simulink model "parfait"  (Simulink 6.0)
settings: Solver=ode23  StartTime=0.0  StopTime=10.0  FixedStep=1e-4  RelTol=1e-3
libraries: simulink x9, aerolibutil x5, aerolibtransform2 x2, mblibv1 x1, aerolib6dof2 x1, vrlib x1
settings Model: LastModifiedBy=sebastien

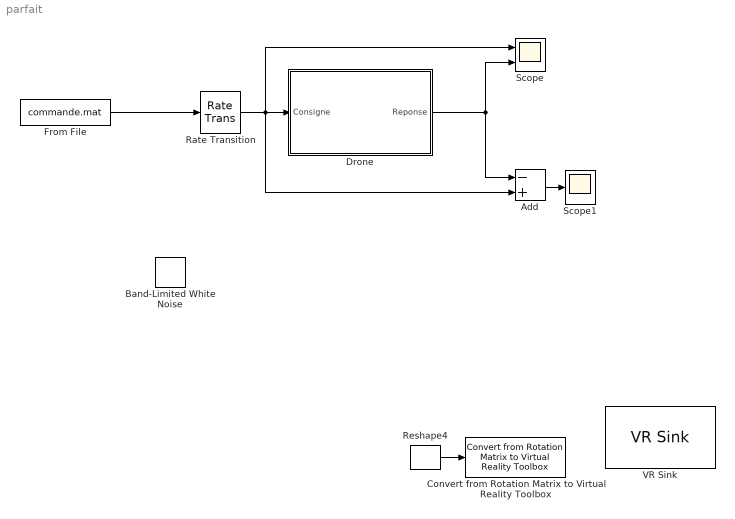
== system parfait ==
  Add : Sum  Inputs=-+  OutScaling=2^-10
  Band-Limited White Noise : simulink/Sources/Band-Limited White Noise  Cov=0.2*[1 1 1 1 1 1]  Ts=1  seed=[23341 3456 665332 234343 232324 45799]
  Convert from Rotation Matrix to Virtual Reality Toolbox : mblibv1/Utilities/Convert from Rotation Matrix to Virtual Reality Toolbox  Tag=Pose2VR
  Drone : Subsystem
  From File : FromFile  FileName=commande.mat  SampleTime=0
  Rate Transition : RateTransition
  Reshape4 : simulink/Math Operations/Reshape  OutputDimensionality=1-D array  OutputDimensions=[1,1]
  Scope : Scope  NumInputPorts=2
      settings: YMin=0~-0.2  YMax=2~2.1
  Scope1 : Scope
  VR Sink : vrlib/VR Sink  SampleTime=0.1  ViewEnable=on  RemoteChange=off  RemoteView=on  FieldsWritten=Drone.center.3.1.double#Drone.rotation.4.1.double  WorldFileName=drone2.WRL  AutoView=off  FigureProperties={}
  wires:
  Reshape4/1 -> Convert from Rotation Matrix to Virtual Reality Toolbox/1
  From File/1 -> Rate Transition/1
  Drone/1(Reponse) -> Scope/2, Add/1
  Rate Transition/1 -> Drone/1(Consigne), Scope/1, Add/2
  Add/1 -> Scope1/1

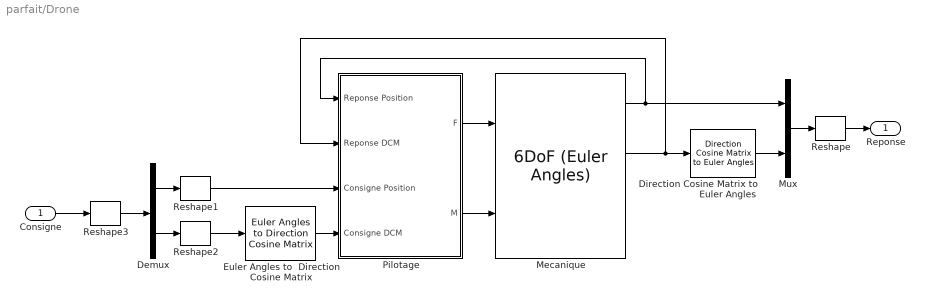
== system parfait/Drone ==
  Consigne : Inport  Port=1  LatchInput=off
  Demux : Demux  Outputs=2
  Direction Cosine Matrix to Euler Angles : aerolibtransform2/Direction Cosine Matrix to Euler Angles
  Euler Angles to  Direction Cosine Matrix : aerolibtransform2/Euler Angles to  Direction Cosine Matrix
  Mecanique : aerolib6dof2/6DoF (Euler Angles)  units=Metric (MKS)  mtype=Fixed  rep=Quaternion  xme_0=[0 0 0]  Vm_0=[0 0 0]  eul_0=[0 0 0]  pm_0=[1 2 4]  mass_0=1.0  mass_e=0  mass_f=0  inertia=eye(3)  inertia_e=eye(3)  inertia_f=eye(3)  k_quat=1.0
  Mux : Mux  Inputs=2
  Pilotage : Subsystem
  Reshape{,1..3} (4 alike) : simulink/Math Operations/Reshape  OutputDimensionality=1-D array  OutputDimensions=[1,1]
  Reponse : Outport
  wires:
  Pilotage/1(F) -> Mecanique/1
  Mecanique/2 -> Pilotage/1(Reponse Position), Mux/1
  Mecanique/4 -> Pilotage/2(Reponse DCM), Direction Cosine Matrix to Euler Angles/1
  Euler Angles to  Direction Cosine Matrix/1 -> Pilotage/4(Consigne DCM)
  Consigne/1 -> Reshape3/1
  Direction Cosine Matrix to Euler Angles/1 -> Mux/2
  Mux/1 -> Reshape/1
  Reshape1/1 -> Pilotage/3(Consigne Position)
  Reshape2/1 -> Euler Angles to  Direction Cosine Matrix/1
  Reshape3/1 -> Demux/1
  Pilotage/2(M) -> Mecanique/2
  Demux/1 -> Reshape1/1
  Demux/2 -> Reshape2/1
  Reshape/1 -> Reponse/1

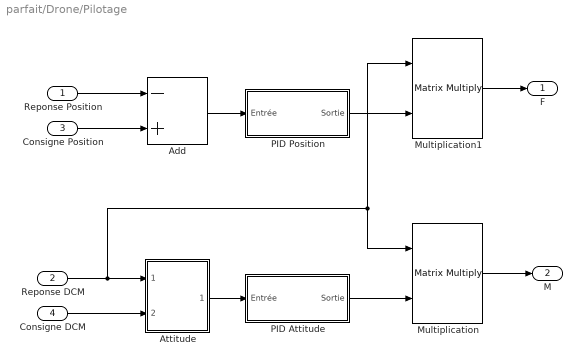
== system parfait/Drone/Pilotage ==
  Reponse Position : Inport  Port=1  LatchInput=off
  Reponse DCM : Inport  Port=2  LatchInput=off
  Consigne Position : Inport  Port=3  LatchInput=off
  Consigne DCM : Inport  Port=4  LatchInput=off
  Add : Sum  Inputs=-+  OutScaling=2^-10  InputSameDT=on
  Attitude : Subsystem
  Multiplication : Product  Inputs=**  Multiplication=Matrix(*)  OutScaling=2^-10
  Multiplication1 : Product  Inputs=**  Multiplication=Matrix(*)  OutScaling=2^-10
  PID Attitude : Subsystem  mask{kp=1000, ki=0.1, kd=0.05, kdd=0}
  PID Position : Subsystem  mask{kp=1000, ki=0.1, kd=0.05, kdd=0}
  F : Outport
  M : Outport  Port=2
  wires:
  Reponse Position/1 -> Add/1
  Consigne Position/1 -> Add/2
  Add/1 -> PID Position/1(Entrée)
  Consigne DCM/1 -> Attitude/2(Consigne)
  Reponse DCM/1 -> Attitude/1(Reponse), Multiplication1/1, Multiplication/1
  Attitude/1(Commande) -> PID Attitude/1(Entrée)
  PID Attitude/1(Sortie) -> Multiplication/2
  PID Position/1(Sortie) -> Multiplication1/2
  Multiplication/1 -> M/1
  Multiplication1/1 -> F/1

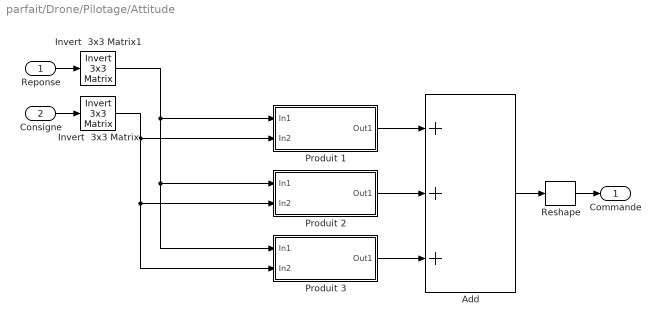
== system parfait/Drone/Pilotage/Attitude ==
  Reponse : Inport  Port=1  LatchInput=off
  Consigne : Inport  Port=2  LatchInput=off
  Add : Sum  Inputs=+++  OutScaling=2^-10
  Invert  3x3 Matrix : aerolibutil/Invert  3x3 Matrix
  Invert  3x3 Matrix1 : aerolibutil/Invert  3x3 Matrix
  Produit 1 : Subsystem  mask{a=[1 0 0]}
      mask prompts: a "Vecteur de reference"
      mask Display: fprintf('Vecteur (%d,%d,%d)', a(1),a(2),a(3))
  Produit 2 : Subsystem  mask{a=[0 1 0]}
      mask prompts: a "Vecteur de reference"
      mask Display: fprintf('Vecteur (%d,%d,%d)', a(1),a(2),a(3))
  Produit 3 : Subsystem  mask{a=[0 0 1]}
      mask prompts: a "Vecteur de reference"
      mask Display: fprintf('Vecteur (%d,%d,%d)', a(1),a(2),a(3))
  Reshape : simulink/Math Operations/Reshape  OutputDimensionality=1-D array  OutputDimensions=[1,1]
  Commande : Outport
  wires:
  Reponse/1 -> Invert  3x3 Matrix1/1
  Consigne/1 -> Invert  3x3 Matrix/1
  Produit 1/1(Out1) -> Add/1
  Produit 2/1(Out1) -> Add/2
  Produit 3/1(Out1) -> Add/3
  Invert  3x3 Matrix/1 -> Produit 1/2(In2), Produit 2/2(In2), Produit 3/2(In2)
  Invert  3x3 Matrix1/1 -> Produit 1/1(In1), Produit 2/1(In1), Produit 3/1(In1)
  Add/1 -> Reshape/1
  Reshape/1 -> Commande/1

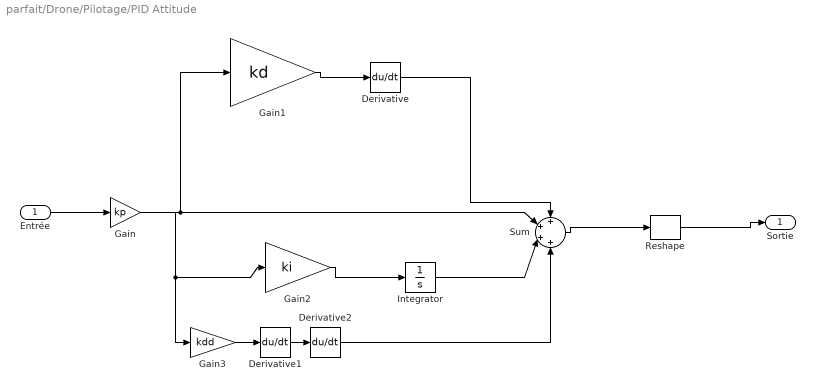
== system parfait/Drone/Pilotage/PID Attitude ==
  Entrée : Inport  Port=1  LatchInput=off
  Derivative : Derivative
  Derivative1 : Derivative
  Derivative2 : Derivative
  Gain : Gain  Gain=kp
  Gain1 : Gain  Gain=kd
  Gain2 : Gain  Gain=ki
  Gain3 : Gain  Gain=kdd
  Integrator : Integrator
  Reshape : simulink/Math Operations/Reshape  OutputDimensionality=1-D array  OutputDimensions=[1,1]
  Sum : Sum  Inputs=++++
  Sortie : Outport
      settings: BusObject=perturbations
  wires:
  Entrée/1 -> Gain/1
  Gain/1 -> Sum/2, Gain1/1, Gain2/1, Gain3/1
  Derivative/1 -> Sum/1
  Integrator/1 -> Sum/3
  Gain2/1 -> Integrator/1
  Gain1/1 -> Derivative/1
  Sum/1 -> Reshape/1
  Gain3/1 -> Derivative1/1
  Derivative1/1 -> Derivative2/1
  Derivative2/1 -> Sum/4
  Reshape/1 -> Sortie/1

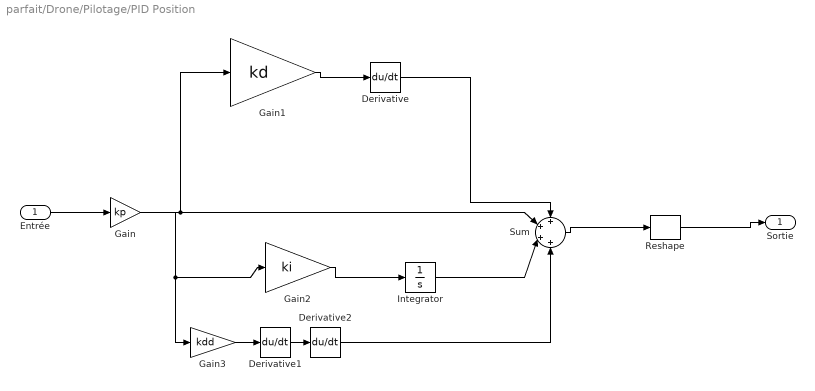
== system parfait/Drone/Pilotage/PID Position ==
  Entrée : Inport  Port=1  LatchInput=off
  Derivative : Derivative
  Derivative1 : Derivative
  Derivative2 : Derivative
  Gain : Gain  Gain=kp
  Gain1 : Gain  Gain=kd
  Gain2 : Gain  Gain=ki
  Gain3 : Gain  Gain=kdd
  Integrator : Integrator
  Reshape : simulink/Math Operations/Reshape  OutputDimensionality=1-D array  OutputDimensions=[1,1]
  Sum : Sum  Inputs=++++
  Sortie : Outport
      settings: BusObject=perturbations
  wires:
  Entrée/1 -> Gain/1
  Gain/1 -> Sum/2, Gain1/1, Gain2/1, Gain3/1
  Derivative/1 -> Sum/1
  Integrator/1 -> Sum/3
  Gain2/1 -> Integrator/1
  Gain1/1 -> Derivative/1
  Sum/1 -> Reshape/1
  Gain3/1 -> Derivative1/1
  Derivative1/1 -> Derivative2/1
  Derivative2/1 -> Sum/4
  Reshape/1 -> Sortie/1

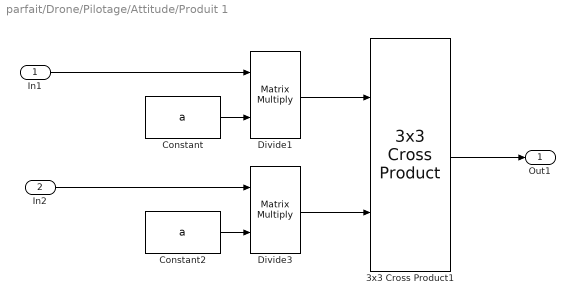
== system parfait/Drone/Pilotage/Attitude/Produit 1 ==
  In1 : Inport  Port=1  LatchInput=off
  In2 : Inport  Port=2  LatchInput=off
  3x3 Cross Product1 : aerolibutil/3x3 Cross Product
  Constant : Constant  Value=a
  Constant2 : Constant  Value=a
  Divide1 : Product  Inputs=**  Multiplication=Matrix(*)  OutScaling=2^-10
  Divide3 : Product  Inputs=**  Multiplication=Matrix(*)  OutScaling=2^-10
  Out1 : Outport
  wires:
  Constant/1 -> Divide1/2
  In1/1 -> Divide1/1
  Constant2/1 -> Divide3/2
  In2/1 -> Divide3/1
  Divide1/1 -> 3x3 Cross Product1/1
  Divide3/1 -> 3x3 Cross Product1/2
  3x3 Cross Product1/1 -> Out1/1

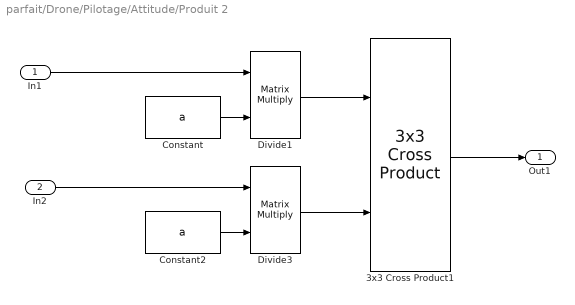
== system parfait/Drone/Pilotage/Attitude/Produit 2 ==
  In1 : Inport  Port=1  LatchInput=off
  In2 : Inport  Port=2  LatchInput=off
  3x3 Cross Product1 : aerolibutil/3x3 Cross Product
  Constant : Constant  Value=a
  Constant2 : Constant  Value=a
  Divide1 : Product  Inputs=**  Multiplication=Matrix(*)  OutScaling=2^-10
  Divide3 : Product  Inputs=**  Multiplication=Matrix(*)  OutScaling=2^-10
  Out1 : Outport
  wires:
  Constant/1 -> Divide1/2
  In1/1 -> Divide1/1
  Constant2/1 -> Divide3/2
  In2/1 -> Divide3/1
  Divide1/1 -> 3x3 Cross Product1/1
  Divide3/1 -> 3x3 Cross Product1/2
  3x3 Cross Product1/1 -> Out1/1

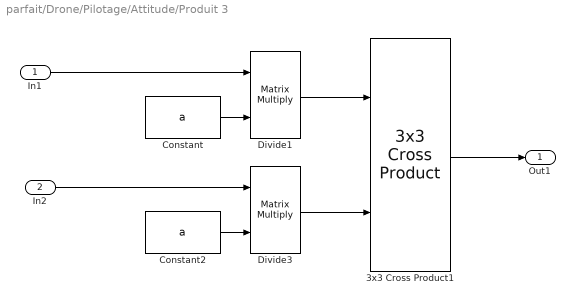
== system parfait/Drone/Pilotage/Attitude/Produit 3 ==
  In1 : Inport  Port=1  LatchInput=off
  In2 : Inport  Port=2  LatchInput=off
  3x3 Cross Product1 : aerolibutil/3x3 Cross Product
  Constant : Constant  Value=a
  Constant2 : Constant  Value=a
  Divide1 : Product  Inputs=**  Multiplication=Matrix(*)  OutScaling=2^-10
  Divide3 : Product  Inputs=**  Multiplication=Matrix(*)  OutScaling=2^-10
  Out1 : Outport
  wires:
  Constant/1 -> Divide1/2
  In1/1 -> Divide1/1
  Constant2/1 -> Divide3/2
  In2/1 -> Divide3/1
  Divide1/1 -> 3x3 Cross Product1/1
  Divide3/1 -> 3x3 Cross Product1/2
  3x3 Cross Product1/1 -> Out1/1
